simulink model "rlc_sim"  (R2018a)
settings: Solver=VariableStepAuto  StartTime=0.0  StopTime=0.1  RelTol=1e-3
Description:
  | 1/C
settings Model: Creator=Dell  LastModifiedBy=user
settings DataIOCC: LimitDataPoints=on  SaveOutput=off  SaveTime=off
settings OptimizationCC: BlockReduction=off  BooleanDataType=off  LifeSpan=inf
settings DebuggingCC: SaveWithParameterizedLinksMsg=none  UnderspecifiedInitializationDetection=Classic  MergeDetectMultiDrivingBlocksExec=none  SignalResolutionControl=TryResolveAllWithWarning  AllowSymbolicDim=off  SFUnexpectedBacktrackingDiag=warning  SFNoUnconditionalDefaultTransitionDiag=warning  SFExecutionAtInitializationDiag=none
settings HardwareCC: TargetUnknown=on
settings CodeAppCC: StateflowObjectComments=on
settings GRTTargetCC: TargetLangStandard=C89/C90 (ANSI)  GeneratePreprocessorConditionals=Disable all

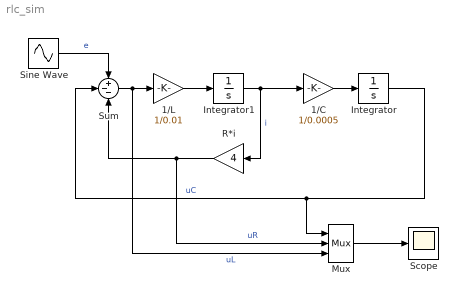
== system rlc_sim ==
  1/C : Gain  Gain=1/0.0005
  1/L : Gain  Gain=1/0.01
  Integrator : Integrator
  Integrator1 : Integrator
  Mux : Mux  Inputs=3
      settings: DisplayOption=signals
  R*i : Gain  Gain=4
  Scope : Scope
  Sine Wave : Sin  Amplitude=sqrt(2)*100  Frequency=314  SampleTime=0.001
  Sum : Sum  Inputs=+--
  wires:
  Integrator/1 -> Mux/1, Sum/2  "uC"
  Sum/1 -> Mux/3, 1/L/1  "uL"
  1/L/1 -> Integrator1/1
  Sine Wave/1 -> Sum/1  "e"
  Integrator1/1 -> R*i/1, 1/C/1  "i"
  Mux/1 -> Scope/1
  R*i/1 -> Mux/2, Sum/3  "uR"
  1/C/1 -> Integrator/1
